simulink model "KF_2018b"  (R2021a)
settings: Solver=FixedStepAuto  StartTime=0.0  StopTime=200  FixedStep=1e-4  RelTol=1e-3
libraries: commchan3 x1
settings Model: Creator=12406  LastModifiedBy=aryal
settings SolverCC: AlgebraicLoopSolver=TrustRegion

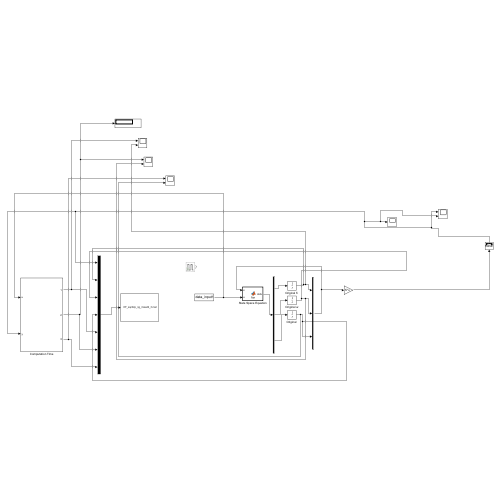
[thumbnail: Simulink's stored preview of the top-level diagram]
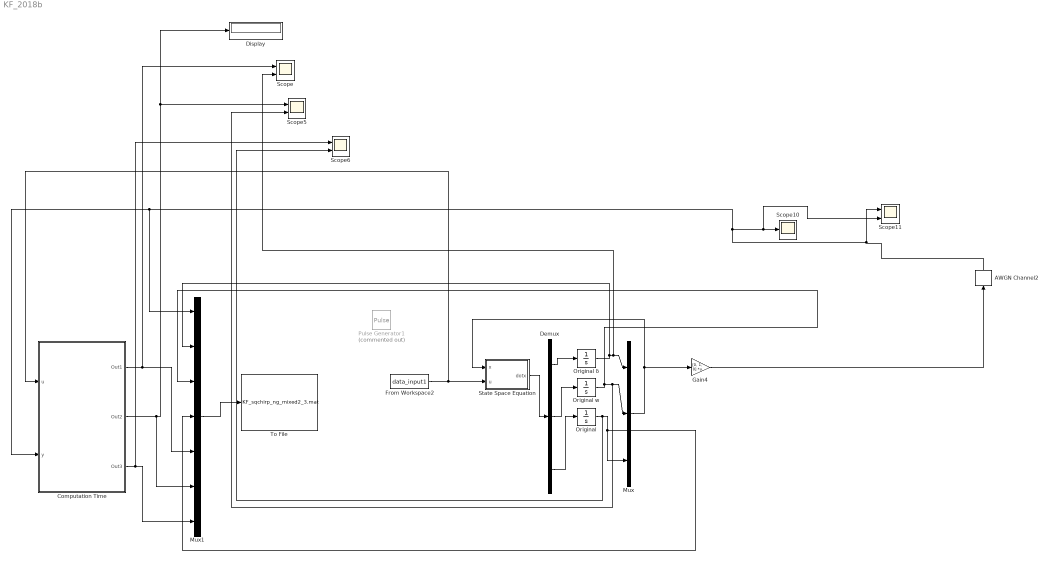
== system KF_2018b ==
  AWGN Channel2 : commchan3/AWGN Channel  InputProcessing=Columns as channels (frame based)  seed=65  noiseMode=Variance from mask  EbNodB=10  EsNodB=10  SNRdB=65  bitsPerSym=1  Ps=1  Tsym=1  variance=1e-6
  Computation Time : Subsystem
  Demux : Demux  Outputs=3
  Display : Display
  From Workspace2 : FromWorkspace  VariableName=data_input1  SampleTime=0.02
  Gain4 : Gain  Gain=[0, 1, 0]  Multiplication=Matrix(K*u)
  Mux : Mux  Inputs=3
  Mux1 : Mux  Inputs=7
  "Original " : Integrator
  Original w : Integrator
  "Original δ " : Integrator
  Pulse Generator1 : DiscretePulseGenerator  Commented=on  PulseType=Time based  Amplitude=0.2  PulseWidth=50
  Scope{,5..6,11} (4 alike) : Scope  NumInputPorts=2
  Scope10 : Scope
  State Space Equation : MATLAB Function  TreatAsAtomicUnit=on
  To File : ToFile  Filename=KF_sqchirp_ng_mixed2_3.mat  MatrixName=w  SampleTime=0.02
  wires:
  Mux/1 -> Gain4/1, State Space Equation/1(x)
  Gain4/1 -> AWGN Channel2/1
  From Workspace2/1 -> Computation Time/1(u), State Space Equation/2(u)
  Original w/1 -> Mux1/3, Scope5/2, Mux/2
  Demux/2 -> Original w/1
  Demux/1 -> "Original δ "/1
  State Space Equation/1(dotx) -> Demux/1
  Demux/3 -> "Original "/1
  "Original "/1 -> Scope6/2, Mux1/4, Mux/3
  Computation Time/1(Out1) -> Scope/1, Mux1/5
  Computation Time/2(Out2) -> Display/1, Scope5/1, Mux1/6
  Computation Time/3(Out3) -> Scope6/1, Mux1/7
  Mux1/1 -> To File/1
  "Original δ "/1 -> Mux1/2, Scope/2, Mux/1
  AWGN Channel2/1 -> Mux1/1, Computation Time/2(y), Scope11/2, Scope10/1, Scope11/1

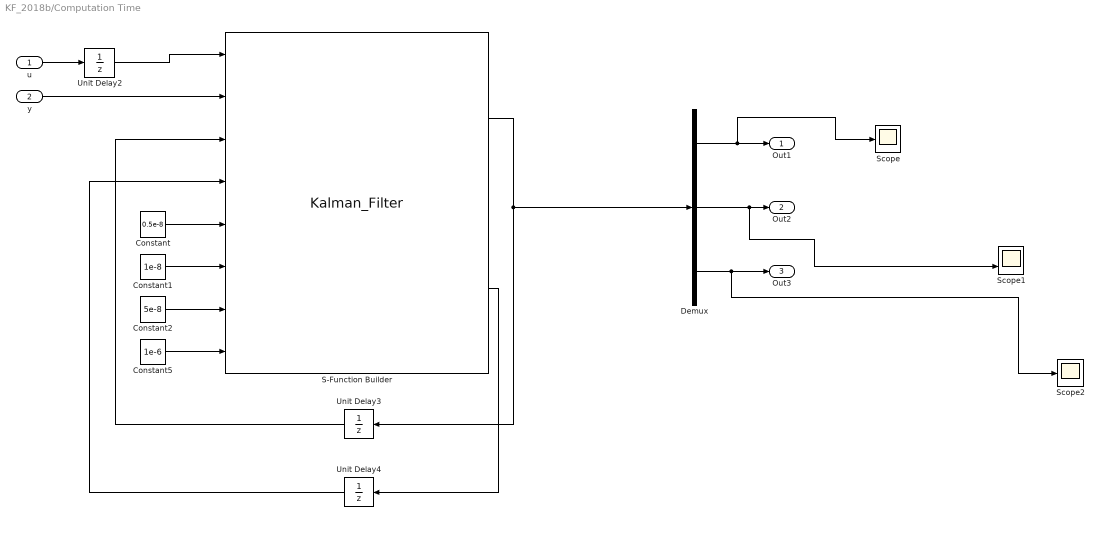
== system KF_2018b/Computation Time ==
  u : Inport
  y : Inport  Port=2
  Constant : Constant  Value=0.5e-8
  Constant1 : Constant  Value=1e-8
  Constant2 : Constant  Value=5e-8
  Constant5 : Constant  Value=1e-6
  Demux : Demux  Outputs=3
  S-Function Builder : S-Function  FunctionName=Kalman_Filter  SFunctionModules=Kalman_Filter_wrapper KF_Code KF_Code_Call  SFunctionDeploymentMode=off  EnableBusSupport=off  mask(S-Function Builder){}
      mask help: Simulink:masks:SFunctionBuilder_MD
      mask init:
      | val = [[.9  0.75 0.75 1 1 .9 .9 1]',[1 1 0.75 0.75 .9 .9 1 .9]'];try , sys = get_param(gcb,'SfunBuilderFcnName');if isempty(sys), sys = get_param(gcb,'FunctionName'); end,catch, sys = get_param(gcb,'FunctionName'); end
      settings: CopyFcn=set_param(gcbh,'LinkStatus','none')  OpenFcn=sfunctionwizard(gcbh)
      mask Display: plot(val(:,1),val(:,2)),disp(sys),port_label('input',1,'u'),port_label('input',2,'y'),port_label('input',3,'xhatp'),port_label('input',4,'Pkp'),port_label('input',5,'Q11'),port_label('input',6,'Q22'),port_label('input',7,'Q33'),port_label('input',8,'R'),port_label('output',1,'xhat'),port_label('output',2,'Pk')
  Scope : Scope
  Scope1 : Scope  NumInputPorts=2
  Scope2 : Scope
  Unit Delay2 : UnitDelay  SampleTime=0.02  HasFrameUpgradeWarning=on
  Unit Delay3 : UnitDelay  InitialCondition=[0;0;0]  SampleTime=0.02  HasFrameUpgradeWarning=on
  Unit Delay4 : UnitDelay  InitialCondition=reshape(diag([10, 10, 10]), 9, 1)  SampleTime=0.02  HasFrameUpgradeWarning=on
  Out1 : Outport
  Out2 : Outport  Port=2
  Out3 : Outport  Port=3
  wires:
  Unit Delay4/1 -> S-Function Builder/4
  Unit Delay3/1 -> S-Function Builder/3
  u/1 -> Unit Delay2/1
  Constant/1 -> S-Function Builder/5
  Constant5/1 -> S-Function Builder/8
  Constant2/1 -> S-Function Builder/7
  S-Function Builder/1 -> Demux/1, Unit Delay3/1
  Constant1/1 -> S-Function Builder/6
  S-Function Builder/2 -> Unit Delay4/1
  Unit Delay2/1 -> S-Function Builder/1
  Demux/1 -> Scope/1, Out1/1
  Demux/2 -> Scope1/2, Out2/1
  Demux/3 -> Scope2/1, Out3/1
  y/1 -> S-Function Builder/2

== matlab function KF_2018b/State Space Equation ==
  data: x input; u input; dotx output
function dotx  = fcn(x, u)
D = 1.5;
M = 4.0;
    Tg = 0.2;
    Rp = 0.05;
    Ki=2;
    dotx = zeros(3, 1);
    x1 = x(1);
    x2 = x(2);
    x3=x(3);
    dotx = [x2;x3;-Ki/(M*Tg)*x1-(D/(M*Tg)+1/(Rp*M*Tg))*x2-(D/M+1/Tg)*x3-1/(M*Tg)*u];
